simulink model "Simulink_Respuesta_Escalon_y_Perturbacion"  (R2020b)
settings: Solver=VariableStepAuto  StartTime=0.0  StopTime=2  RelTol=1e-3
values from neighbouring files (symbols this model uses):
  Amplitud_referencia = 1    [Contolador_Por_Modelo_Interno.m]
  KM = 1    [Contolador_Por_Modelo_Interno.m]
  TaoF = TaoM/2    (= 0.025)    [Contolador_Por_Modelo_Interno.m]
  TaoM = 0.05    [Contolador_Por_Modelo_Interno.m]
  Tiempo_escalon = 0.5    [Contolador_Por_Modelo_Interno.m]
  TL = 0.1    [Contolador_Por_Modelo_Interno.m]
undefined symbols (not defined in the file or in its folder): sigbuilder_block
settings Model: Creator=Fernando Madera  LastModifiedBy=Fernando Madera

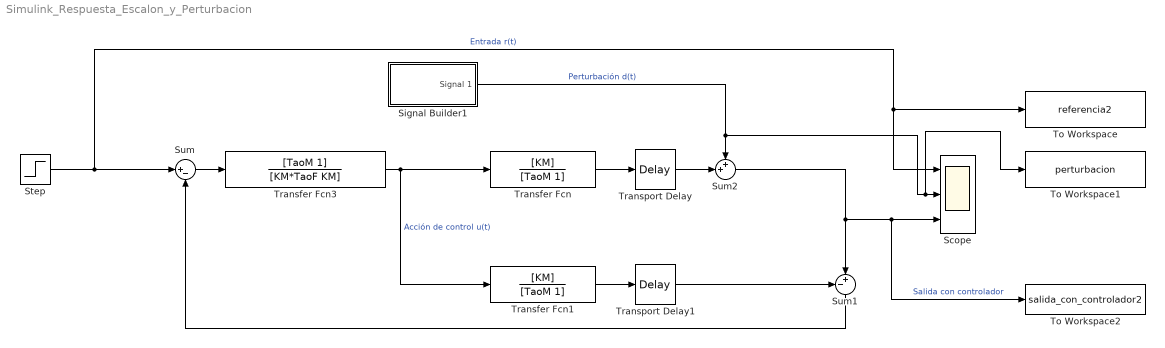
== system Simulink_Respuesta_Escalon_y_Perturbacion ==
  Scope : Scope  NumInputPorts=3
  Signal Builder1 : Subsystem  Tag=STV Subsys  LoadFcn=sigbuilder_block('load');  StartFcn=sigbuilder_block('start');  StopFcn=sigbuilder_block('stop');  ClipboardFcn=sigbuilder_block('clipboard');  mask(Sigbuilder block){tuvar=[0:10]}
      mask help: Simulink:masks:SigbuilderBlock_MD
      mask init:
      | if ~strcmp(get_param(bdroot(gcbh),'SimulationStatus'),'stopped') tuvar = sigbuilder_block('maskInit'); end
      settings: CopyFcn=sigbuilder_block('copy');  DeleteFcn=sigbuilder_block('delete');  ModelCloseFcn=sigbuilder_block('modelClose');  PreSaveFcn=sigbuilder_block('preSave');  PauseFcn=sigbuilder_block('pause');  ContinueFcn=sigbuilder_block('continue');  NameChangeFcn=sigbuilder_block('namechange');  OpenFcn=sigbuilder_block('open',[5.5 30 949 418 ]);  CloseFcn=sigbuilder_block('close');
      mask Display: plot(0, 0, 100, 100,[2, 2, 32, 32, 2], [68, 8, 8, 68, 68],[32, 2], [38, 38], [32, 19, 2],[53, 60, 44], [32, 17, 17, 2],[16, 16, 31, 31]);txt = getActiveGroup(gcbh);text(2, 100, txt,'verticalAlignment', 'top');
  Step : Step  Time=Tiempo_escalon  After=Amplitud_referencia  SampleTime=0
  Sum : Sum  Inputs=|+-
  Sum1 : Sum  Inputs=-+|
  Sum2 : Sum  Inputs=++|
  To Workspace : ToWorkspace  VariableName=referencia2  SaveFormat=Timeseries  SampleTime=-1
  To Workspace1 : ToWorkspace  VariableName=perturbacion  SaveFormat=Timeseries  SampleTime=-1
  To Workspace2 : ToWorkspace  VariableName=salida_con_controlador2  SaveFormat=Timeseries  SampleTime=-1
  Transfer Fcn : TransferFcn  Numerator=[KM]  Denominator=[TaoM 1]
  Transfer Fcn1 : TransferFcn  Numerator=[KM]  Denominator=[TaoM 1]
  Transfer Fcn3 : TransferFcn  Numerator=[TaoM 1]  Denominator=[KM*TaoF KM]
  Transport Delay : TransportDelay  DelayTime=TL
  Transport Delay1 : TransportDelay  DelayTime=TL
  wires:
  Transfer Fcn3/1 -> Transfer Fcn/1, Transfer Fcn1/1  "Acción de control u(t)"
  Sum2/1 -> To Workspace2/1, Scope/3, Sum1/2  "Salida con controlador"
  Transfer Fcn/1 -> Transport Delay/1
  Transport Delay1/1 -> Sum1/1
  Transfer Fcn1/1 -> Transport Delay1/1
  Sum1/1 -> Sum/2
  Sum/1 -> Transfer Fcn3/1
  Step/1 -> Scope/1, To Workspace/1, Sum/1  "Entrada r(t)"
  Signal Builder1/1(Signal 1) -> To Workspace1/1, Scope/2, Sum2/1  "Perturbación d(t)"
  Transport Delay/1 -> Sum2/2

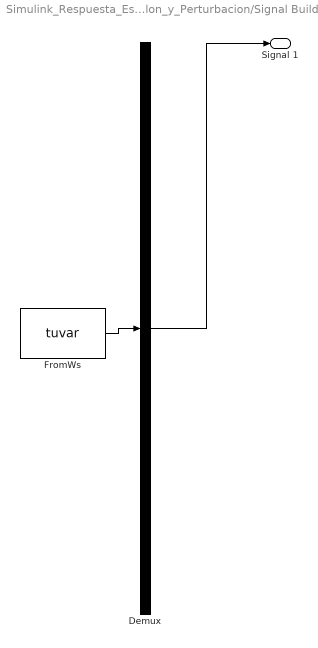
== system Simulink_Respuesta_Escalon_y_Perturbacion/Signal Builder1 ==
  Demux : Demux  Tag=STV Demux  Outputs=1
      settings: DisplayOption=none
  FromWs : FromWorkspace  Tag=STV FromWs  VariableName=tuvar
      SigBuilderData=|
      | common.afterFinalStr = 'Extrapolate'
      | common.sampleTime = 0
      | dataSet.timeRange = [0 2]
      | dataSet.name = 'Group 1'
      | sbobj.Groups.Name = 'Group 1'
      | sbobj.Groups.Signals.Name = 'Signal 1'
      | sbobj.Groups.Signals.XData = [0 1.2 1.2 1.25 1.25 2]
      | sbobj.Groups.Signals.YData = [0 0 0.5 0.5 0 0]
      | sbobj.Groups.TimeRange = [0 2]
  Signal 1 : Outport  Tag=STV Outport
  wires:
  FromWs/1 -> Demux/1
  Demux/1 -> Signal 1/1
